simulink model "MSFartoystyring"  (R2019a)
settings: Solver=ode45  StartTime=tstart  StopTime=tstop  RelTol=1e-3  EnableMultiTasking=on
values from neighbouring files (symbols this model uses):
  c = 1    [run.m]
  delta_max = deg2rad(25)    [defines.m]
  K_psi = r_inf / (-delta_max * T_psi)    [defines.m]
  L_pp = 304.8    [defines.m]
  p0 = zeros(2,1)    [run.m]
  psi0 = 0    [run.m]
  r0 = 0    [run.m]
  T_psi = 140    [defines.m]
  tsamp = 10    [run.m]
  v0 = [6.63 0]'    [run.m]
undefined symbols (not defined in the file or in its folder): heading_controller, msfartoystyring
settings Model: ExtModeAutoUpdateStatusClock=off  Creator=christh  LastModifiedBy=martiege
settings DataIOCC: LimitDataPoints=on  SaveFormat=Array  SignalLoggingSaveFormat=ModelDataLogs  ReturnWorkspaceOutputs=off
settings OptimizationCC: ExpressionDepthLimit=2147483647  InitFltsAndDblsToZero=on  LifeSpan=inf
settings DebuggingCC: UnderspecifiedInitializationDetection=Classic  MergeDetectMultiDrivingBlocksExec=none  SolverPrmCheckMsg=warning  FcnCallInpInsideContextMsg=warning  StateNameClashWarn=warning  SFUnexpectedBacktrackingDiag=warning  SFNoUnconditionalDefaultTransitionDiag=warning  ArithmeticOperatorsInVariantConditions=warning
settings HardwareCC: ProdBitPerPointer=32  ProdBitPerSizeT=32  ProdBitPerPtrDiffT=32  ProdLargestAtomicFloat=None  ProdIntDivRoundTo=Undefined  ProdEndianess=Unspecified  ProdWordSize=32  ProdHWDeviceType=32-bit Generic
settings ModelReferenceCC: PropagateSignalLabelsOutOfModel=off
settings SFSimCC: SimUseLocalCustomCode=off
settings RTWCC: RTWUseLocalCustomCode=off
settings CodeAppCC: StateflowObjectComments=on
settings GRTTargetCC: TargetLangStandard=C89/C90 (ANSI)  GeneratePreprocessorConditionals=Disable all  CombineOutputUpdateFcns=off  GRTInterface=on
settings ConfigComp: CovMetricSettings=dw  CovHtmlReporting=on  CovSaveCumulativeToWorkspaceVar=on  CovSaveSingleToWorkspaceVar=on  CovExternalEMLEnable=off

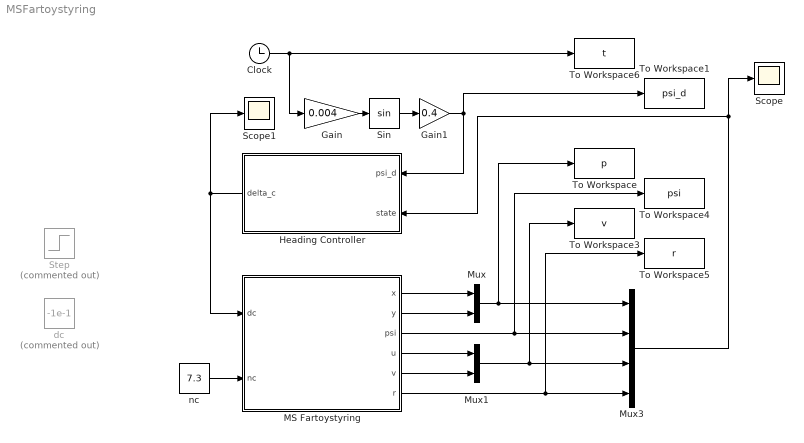
== system MSFartoystyring ==
  Clock : Clock
  Gain : Gain  Gain=0.004
  Gain1 : Gain  Gain=0.4
  "Heading Controller " : Subsystem
  MS Fartoystyring : Subsystem  mask(MS Fartoystyring for Assignment 3 G&C){x0=p0(1), y0=p0(2), u0=v0(1), v0=v0(2), psi0=psi0, r0=r0, c=c}
      mask prompts: x0 "x(t0) (m)"; y0 "y(t0) (m)"; u0 "u(t0) (m/s)"; v0 "v(t0) (m/s)"; psi0 "psi(t0) (rad)"; r0 "r(t0) (rad/s)"; c "current (0 or 1)"
      mask help:
      | Block corresponding to Figure 1 in the assignment text. Gives the response of the ship.
      |
      | The design speed of MS Fartoystyring is u=8.23 m/s.
      |
      | Input:
      | dc: commanded rudder (rad), dmax=25*pi/180
      | nc: commanded shaft speed (rad/s), nmax=85*2*pi/60
      |
      | Output:
      | x: north pos (m)
      | y: east pos (m)
      | u: surge (m/s)
      | v: sway (m/s)
      | psi: heading (rad)
      | r: yaw (rad/s)
      mask Help: Comments, bugs and help requests can be directed to the TA. Email on course website.
  Mux : Mux  Inputs=2
  Mux1 : Mux  Inputs=2
  Mux3 : Mux
  Scope : Scope
  Scope1 : Scope
  Sin : Trigonometry
  Step : Step  Commented=on  Time=0  After=-deg2rad(25)  SampleTime=0
  To Workspace : ToWorkspace  VariableName=p  SampleTime=tsamp
  To Workspace1 : ToWorkspace  VariableName=psi_d  SampleTime=tsamp
  To Workspace3 : ToWorkspace  VariableName=v  SampleTime=tsamp
  To Workspace4 : ToWorkspace  VariableName=psi  SampleTime=tsamp
  To Workspace5 : ToWorkspace  VariableName=r  SampleTime=tsamp
  To Workspace6 : ToWorkspace  VariableName=t  SampleTime=tsamp
  dc : Constant  Commented=on  Value=-1e-1
  nc : Constant  Value=7.3
  wires:
  Clock/1 -> To Workspace6/1, Gain/1
  MS Fartoystyring/1(x) -> Mux/1
  MS Fartoystyring/2(y) -> Mux/2
  MS Fartoystyring/4(u) -> Mux1/1
  MS Fartoystyring/5(v) -> Mux1/2
  Mux/1 -> To Workspace/1, Mux3/1
  Mux1/1 -> To Workspace3/1, Mux3/3
  MS Fartoystyring/3(psi) -> To Workspace4/1, Mux3/2
  MS Fartoystyring/6(r) -> To Workspace5/1, Mux3/4
  nc/1 -> MS Fartoystyring/2(nc)
  Mux3/1 -> "Heading Controller "/2(state), Scope/1
  "Heading Controller "/1(delta_c) -> Scope1/1, MS Fartoystyring/1(dc)
  Gain/1 -> Sin/1
  Sin/1 -> Gain1/1
  Gain1/1 -> "Heading Controller "/1(psi_d), To Workspace1/1

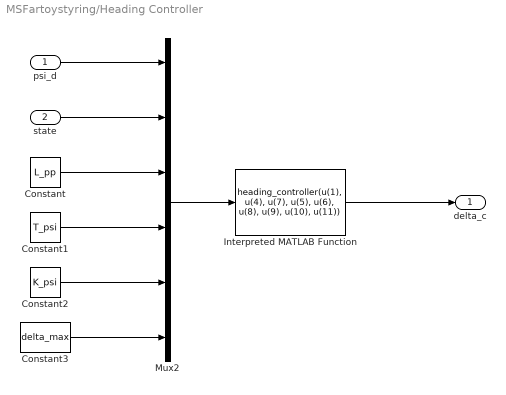
== system MSFartoystyring/Heading Controller  ==
  psi_d : Inport
  state : Inport  Port=2
  Constant : Constant  Value=L_pp
  Constant1 : Constant  Value=T_psi
  Constant2 : Constant  Value=K_psi
  Constant3 : Constant  Value=delta_max
  Interpreted MATLAB Function : MATLABFcn  MATLABFcn=heading_controller(u(1), u(4), u(7), u(5), u(6), u(8), u(9), u(10), u(11))
  Mux2 : Mux  Inputs=6
  delta_c : Outport
  wires:
  Constant3/1 -> Mux2/6
  Constant/1 -> Mux2/3
  psi_d/1 -> Mux2/1
  Constant1/1 -> Mux2/4
  state/1 -> Mux2/2
  Interpreted MATLAB Function/1 -> delta_c/1
  Mux2/1 -> Interpreted MATLAB Function/1
  Constant2/1 -> Mux2/5

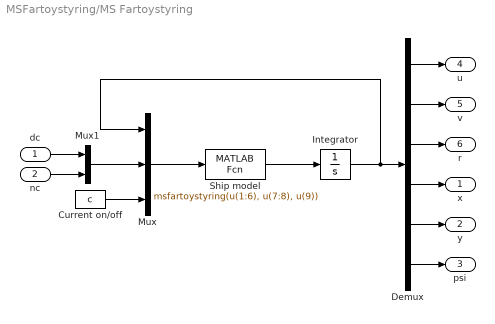
== system MSFartoystyring/MS Fartoystyring ==
  dc : Inport
  nc : Inport  Port=2
  Current on/off : Constant  Value=c
  Demux : Demux  Outputs=6
  Integrator : Integrator  InitialCondition=[u0 v0 r0 x0 y0 psi0]'
  Mux : Mux  Inputs=3
  Mux1 : Mux  Inputs=2
  Ship model : MATLABFcn  MATLABFcn=msfartoystyring(u(1:6), u(7:8), u(9))  OutputDimensions=6
  x : Outport
  y : Outport  Port=2
  psi : Outport  Port=3
  u : Outport  Port=4
  v : Outport  Port=5
  r : Outport  Port=6
  wires:
  Integrator/1 -> Mux/1, Demux/1
  Mux1/1 -> Mux/2
  dc/1 -> Mux1/1
  nc/1 -> Mux1/2
  Demux/1 -> u/1
  Demux/2 -> v/1
  Demux/3 -> r/1
  Demux/4 -> x/1
  Demux/5 -> y/1
  Demux/6 -> psi/1
  Current on/off/1 -> Mux/3
  Ship model/1 -> Integrator/1
  Mux/1 -> Ship model/1
